simulink model "BO_DK_PI_MO_HE_ROBOT_2_DOF"  (R2017b)
settings: Solver=FixedStepAuto  StartTime=0.0  StopTime=40  FixedStep=0.01  RelTol=1e-3
libraries: fuzblock x2
settings Model: Creator=ASUS  LastModifiedBy=DELL
settings SFSimCC: SimUseLocalCustomCode=on
settings RTWCC: RTWUseLocalCustomCode=on
settings CodeAppCC: StateflowObjectComments=on

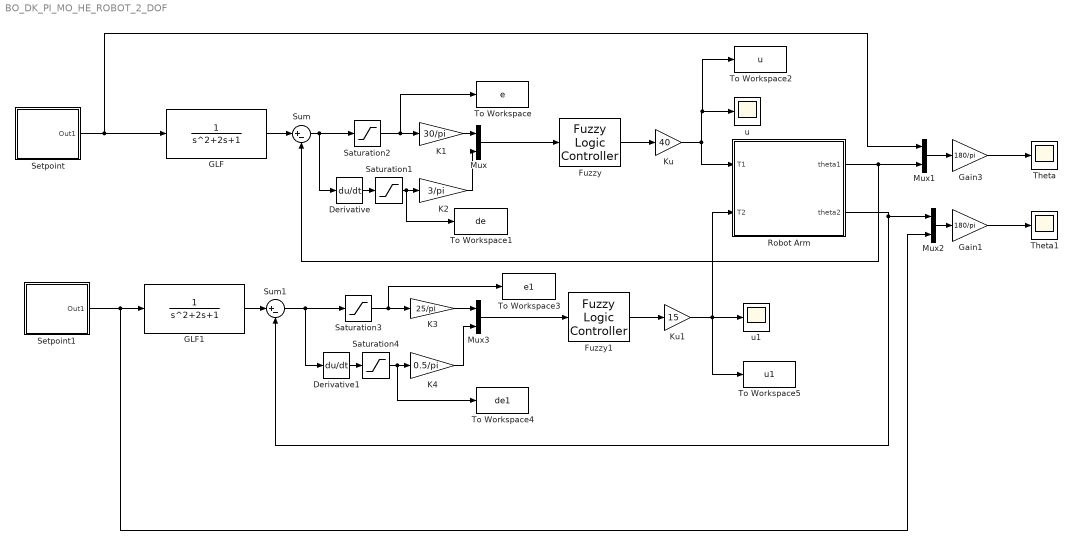
== system BO_DK_PI_MO_HE_ROBOT_2_DOF ==
  Derivative : Derivative
  Derivative1 : Derivative
  Fuzzy : fuzblock/Fuzzy Logic  Controller  FIS="\"Sugenofuzzyrobot.fis\""  OutputSampleNumber=101  DataType=double  FuzzifiedInputs=off  RuleFiringStrengths=off  RuleOutputs=off  AggregatedOutputs=off  SimulateUsing=Interpreted execution
  Fuzzy1 : fuzblock/Fuzzy Logic  Controller  FIS="\"Sugenofuzzyrobot.fis\""  OutputSampleNumber=101  DataType=double  FuzzifiedInputs=off  RuleFiringStrengths=off  RuleOutputs=off  AggregatedOutputs=off  SimulateUsing=Interpreted execution
  GLF : TransferFcn
  GLF1 : TransferFcn
  Gain1 : Gain  Gain=180/pi
  Gain3 : Gain  Gain=180/pi
  K1 : Gain  Gain=30/pi
  K2 : Gain  Gain=3/pi
  K3 : Gain  Gain=25/pi
  K4 : Gain  Gain=0.5/pi
  Ku : Gain  Gain=40
  Ku1 : Gain  Gain=15
  Mux{,1..3} (4 alike) : Mux  Inputs=2
  Robot Arm : Subsystem
  Saturation{1..4} (4 alike) : Saturate  UpperLimit=1  LowerLimit=-1
  Setpoint : Subsystem
  Setpoint1 : Subsystem
  Sum : Sum  Inputs=|+-
  Sum1 : Sum  Inputs=|+-
  Theta : Scope
  Theta1 : Scope
  To Workspace : ToWorkspace  VariableName=e  SampleTime=-1
  To Workspace1 : ToWorkspace  VariableName=de  SampleTime=-1
  To Workspace2 : ToWorkspace  VariableName=u  SampleTime=-1
  To Workspace3 : ToWorkspace  VariableName=e1  SampleTime=-1
  To Workspace4 : ToWorkspace  VariableName=de1  SampleTime=-1
  To Workspace5 : ToWorkspace  VariableName=u1  SampleTime=-1
  u : Scope
  u1 : Scope
  wires:
  Sum/1 -> Derivative/1, Saturation2/1
  K2/1 -> Mux/2
  Mux/1 -> Fuzzy/1
  Fuzzy/1 -> Ku/1
  Ku/1 -> Robot Arm/1(T1), To Workspace2/1, u/1
  Robot Arm/1(theta1) -> Mux1/2, Sum/2
  Mux1/1 -> Gain3/1
  Gain3/1 -> Theta/1
  Setpoint/1(Out1) -> GLF/1, Mux1/1
  Gain1/1 -> Theta1/1
  Mux2/1 -> Gain1/1
  Robot Arm/2(theta2) -> Mux2/1, Sum1/2
  Fuzzy1/1 -> Ku1/1
  Mux3/1 -> Fuzzy1/1
  Ku1/1 -> To Workspace5/1, u1/1, Robot Arm/2(T2)
  GLF/1 -> Sum/1
  Setpoint1/1(Out1) -> Mux2/2, GLF1/1
  GLF1/1 -> Sum1/1
  K1/1 -> Mux/1
  K3/1 -> Mux3/1
  K4/1 -> Mux3/2
  Saturation2/1 -> To Workspace/1, K1/1
  Saturation1/1 -> To Workspace1/1, K2/1
  Derivative/1 -> Saturation1/1
  Sum1/1 -> Saturation3/1, Derivative1/1
  Saturation3/1 -> To Workspace3/1, K3/1
  Derivative1/1 -> Saturation4/1
  Saturation4/1 -> To Workspace4/1, K4/1

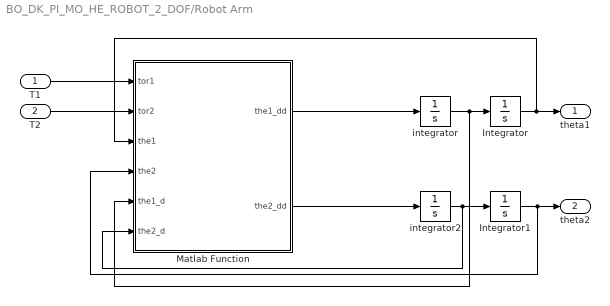
== system BO_DK_PI_MO_HE_ROBOT_2_DOF/Robot Arm ==
  T1 : Inport
  T2 : Inport  Port=2
  Integrator : Integrator
  Integrator1 : Integrator
  Matlab Function : MATLAB Function  TreatAsAtomicUnit=on
  integrator : Integrator
  integrator2 : Integrator
  theta1 : Outport
  theta2 : Outport  Port=2
  wires:
  Integrator/1 -> Matlab Function/3(the1), theta1/1
  integrator/1 -> Matlab Function/5(the1_d), Integrator/1
  Matlab Function/1(the1_dd) -> integrator/1
  Matlab Function/2(the2_dd) -> integrator2/1
  integrator2/1 -> Matlab Function/6(the2_d), Integrator1/1
  Integrator1/1 -> Matlab Function/4(the2), theta2/1
  T1/1 -> Matlab Function/1(tor1)
  T2/1 -> Matlab Function/2(tor2)

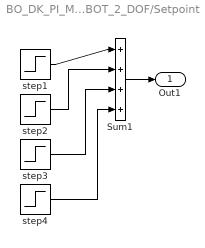
== system BO_DK_PI_MO_HE_ROBOT_2_DOF/Setpoint ==
  Sum1 : Sum  Inputs=|++++
  step1 : Step  Time=0  After=-pi/4  SampleTime=0
  step2 : Step  Time=10  After=pi/4  SampleTime=0
  step3 : Step  Time=20  After=-pi/6  SampleTime=0
  step4 : Step  Time=30  After=pi/3  SampleTime=0
  Out1 : Outport
  wires:
  step1/1 -> Sum1/1
  step2/1 -> Sum1/2
  step4/1 -> Sum1/4
  step3/1 -> Sum1/3
  Sum1/1 -> Out1/1

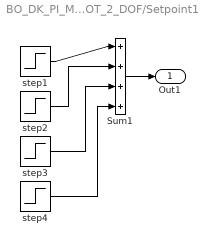
== system BO_DK_PI_MO_HE_ROBOT_2_DOF/Setpoint1 ==
  Sum1 : Sum  Inputs=|++++
  step1 : Step  Time=0  After=pi/6  SampleTime=0
  step2 : Step  Time=10  After=-pi/3  SampleTime=0
  step3 : Step  Time=20  After=pi/6  SampleTime=0
  step4 : Step  Time=30  After=-pi/4  SampleTime=0
  Out1 : Outport
  wires:
  Sum1/1 -> Out1/1
  step3/1 -> Sum1/3
  step4/1 -> Sum1/4
  step2/1 -> Sum1/2
  step1/1 -> Sum1/1

== matlab function BO_DK_PI_MO_HE_ROBOT_2_DOF/Robot Arm/Matlab Function ==
  data: tor1 input; tor2 input; the1_dd output; the1 input; the2 input; the1_d input; the2_d input; the2_dd output
function [the1_dd,the2_dd] = PTVP(tor1,tor2,the1,the2,the1_d,the2_d)
J1=0.05;
J2=0.05;
m1=1;
m2=1;
m3=0;%Khoi luong cua hai khop
l1=1;
l2=1;
lc1=0.4;
lc2=0.4;
g=9.81;
H11=J1+J2+m1*(lc1^2)+m2*((l1^2)+(lc2^2)+2*l1*lc2*cos(the2))+m3*(l1*l1+l2*l2+2*l1*l2*cos(the2));
H22=J2+m2*lc2*lc2+m3*l2*l2;
H12=J2+m2*(lc2*lc2+l1*lc2*cos(the2))+m3*(l2*l2+2*l1*l2*cos(the2));
H21=H12;
H=[H11 H12;
   H21 H22];
h=m2*l1*lc2*sin(the2);

V=[-h*the2_d   -h*the1_d - h*the2_d;
   -h*the1_d    0];
g1=m1*lc1*g*cos(the1)+m2*g*(lc2*cos(the1+the2)+l1*cos(the1));
g2=m2*lc2*g*cos(the1+the2);
G=[g1;
    g2];
tor=[tor1;
     tor2;];
the_dd=pinv(H)*(tor-G-V*[the1_d;the2_d]);
%-diag([1;1])*[the1_d;the2_d]
the1_dd=the_dd(1);
the2_dd=the_dd(2);
end
